simulink library "three_chessclock_library"  (R2018b)
settings: Solver=VariableStepAuto  StartTime=0.0  StopTime=10.0  RelTol=1e-3
settings Model: Creator=svdh  LastModifiedBy=svdh

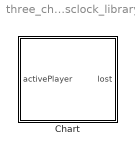
== system three_chessclock_library ==
  Chart : Stateflow chart  TreatAsAtomicUnit=on

== stateflow chart three_chessclock_library/Chart ==
  state ChessClock [parallel]
    settings: executionOrder=1
    state Active
      state localTick
      state localTock
        entry:
        localT = localT - 1
      state globalTick
      state globalTock
        entry:
        globalT = globalT -1
      state Boom
        lost = 1
      (default) -> localTick
      localTick -> localTock : after(1,sec)
      localTock -> localTick [order 2] : [localT > 0]
      localTock -> globalTick [order 1] : [localT == 0]
      globalTick -> globalTock : after(1,sec)
      globalTock -> globalTick [order 1] : [globalT > 0]
      globalTock -> Boom [order 2] : [globalT == 0]
    state Inactive
      entry:
      localT = 10
      globalT = globalT + 15
    (default) -> Inactive : {globalT = (60*30) - 15; lost = 0}
    Active -> Inactive : [activePlayer == 0]
    Inactive -> Active : [activePlayer == 1]
  state addTime [parallel]
    settings: executionOrder=2
    state moveCounter
    state incrementMoves
      entry:
      moves = moves + 1
    state addingTime
      entry:
      globalT = globalT + (15*60)
    (default) -> moveCounter : {moves = 0}
    moveCounter -> incrementMoves [order 2] : [activePlayer == 1]
    incrementMoves -> moveCounter : [activePlayer == 0]
    moveCounter -> addingTime [order 1] : [moves == 40]
  data: globalT local; activePlayer input; localT local; moves local; lost output
